simulink model "RCS_Model"  (R2023a)
settings: Solver=VariableStepAuto  StartTime=0.0  StopTime=tf  RelTol=1e-3
undefined symbols (not defined in the file or in its folder): eom_rcs, rcs
settings Model: Creator=User  LastModifiedBy=User

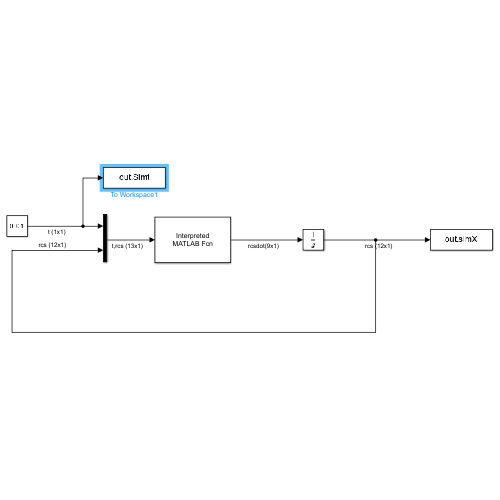
[thumbnail: Simulink's stored preview of the top-level diagram]
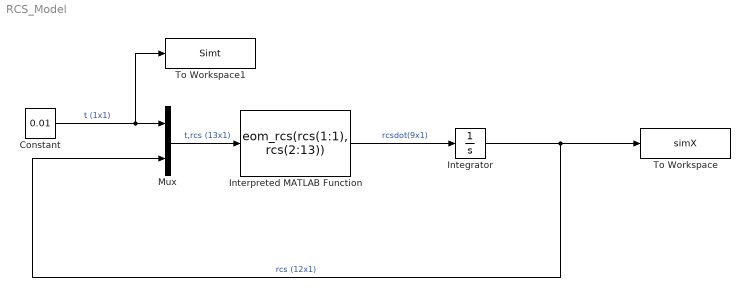
== system RCS_Model ==
  Constant : Constant  Value=0.01
  Integrator : Integrator
  Interpreted MATLAB Function : MATLABFcn  MATLABFcn=eom_rcs(rcs(1:1), rcs(2:13))  Output1D=off
  Mux : Mux  Inputs=2
  To Workspace : ToWorkspace  VariableName=simX  SaveFormat=Timeseries  SampleTime=-1
  To Workspace1 : ToWorkspace  VariableName=Simt  SaveFormat=Timeseries  SampleTime=-1
  wires:
  Interpreted MATLAB Function/1 -> Integrator/1  "rcsdot(9x1)"
  Integrator/1 -> To Workspace/1, Mux/2  "rcs (12x1)"
  Constant/1 -> To Workspace1/1, Mux/1  "t (1x1)"
  Mux/1 -> Interpreted MATLAB Function/1  "t,rcs (13x1)"
